simulink model "simulink8"  (R2023a)
settings: Solver=VariableStepAuto  StartTime=0.0  StopTime=10.0  MaxStep=0.0001  RelTol=1e-3
values from neighbouring files (symbols this model uses):
  Kt = 0.01    [ElecMec.m]
  Kv = 0.01    [ElecMec.m]
  L = 23e-3    (= 0.023)    [ElecMec.m]
  R = 2    [ElecMec.m]
undefined symbols (not defined in the file or in its folder): b, j
settings Model: Creator=maria  LastModifiedBy=erick

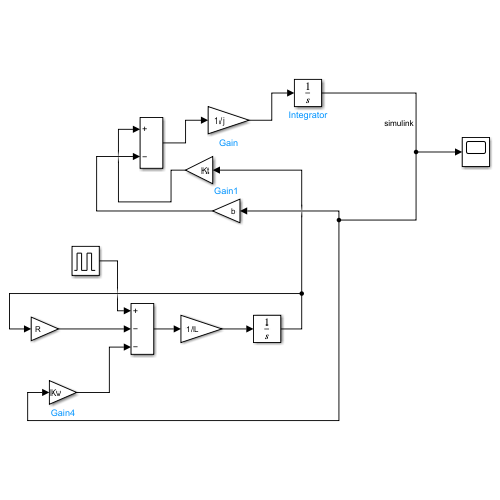
[thumbnail: Simulink's stored preview of the top-level diagram]
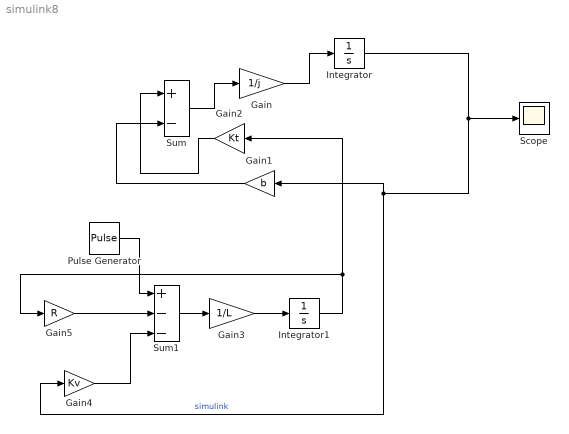
== system simulink8 ==
  Gain : Gain  Gain=1/j
  Gain1 : Gain  Gain=b
  Gain2 : Gain  Gain=Kt
  Gain3 : Gain  Gain=1/L
  Gain4 : Gain  Gain=Kv
  Gain5 : Gain  Gain=R
  Integrator : Integrator
  Integrator1 : Integrator
  Pulse Generator : DiscretePulseGenerator  PulseType=Time based  Amplitude=24  Period=1/2000  PulseWidth=21
  Scope : Scope
  Sum : Sum  Inputs=+-
  Sum1 : Sum  Inputs=+--
  wires:
  Integrator/1 -> Gain4/1, Gain1/1, Scope/1  "simulink"
  Sum/1 -> Gain/1
  Gain/1 -> Integrator/1
  Gain1/1 -> Sum/2
  Gain2/1 -> Sum/1
  Sum1/1 -> Gain3/1
  Gain3/1 -> Integrator1/1
  Gain4/1 -> Sum1/3
  Gain5/1 -> Sum1/2
  Pulse Generator/1 -> Sum1/1
  Integrator1/1 -> Gain5/1, Gain2/1
